simulink model "torqueBalancingYogaWithQPBlock2017a_"  (Simulink 8.9)
settings: Solver=FixedStepDiscrete  StartTime=0.0  StopTime="Config.SIMULATION_TIME "  FixedStep=Config.Ts  RelTol=1e-3  EnableMultiTasking=on
InitFcn:
  | cd(fileparts(which(bdroot)));
  | initTorqueBalancingYoga;
StopFcn:
  | cd(fileparts(which(bdroot)));
  | stopTorqueBalancingYoga;
undefined symbols (not defined in the file or in its folder): bVectorConstraints, Config, ConstraintsMatrix, Gain, Reg, ROBOT_DOF, ROBOT_DOF_FOR_SIMULINK, Sat, Sm
libraries: WBToolboxLibrary x90, simulink x4
(part 1 of 2)
settings Model: SuppressorTable=22 serialization::archive 11 0 6 0 0 0 1 0  Creator=daniele  LastModifiedBy=root
settings DataIOCC: SignalLoggingSaveFormat=Dataset
settings OptimizationCC: ExpressionDepthLimit=2147483647
settings DebuggingCC: SolverPrmCheckMsg=warning  AllowSymbolicDim=off
settings SFSimCC: SimParseCustomCode=off
settings RTWCC: GenCodeOnly=on  RetainRTWFile=on  BuildConfiguration=Debug  TargetLang=C++
settings GRTTargetCC: TargetLangStandard=C++03 (ISO)  GenerateFullHeader=off  CombineOutputUpdateFcns=on  MatFileLogging=off  MultiInstanceERTCode=on  CodeInterfacePackaging=C++ class  SupportNonFinite=off  GRTInterface=off
settings CPPComponent: GenerateDestructor=on  GenerateExternalIOAccessMethods=None  ParameterMemberVisibility=private  InternalMemberVisibility=private  GenerateParameterAccessMethods=None  GenerateInternalMemberAccessMethods=None  UseOperatorNewForModelRefRegistration=off

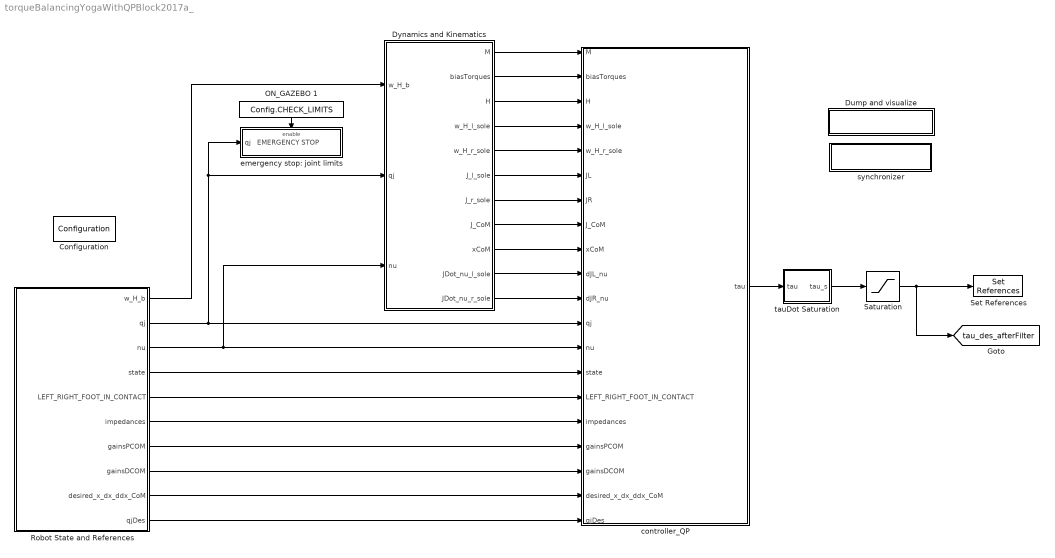
== system torqueBalancingYogaWithQPBlock2017a_ ==
  Configuration : WBToolboxLibrary/Utilities/Configuration  ConfigSource=Workspace  ConfigObject='WBTConfigRobot'
      settings: SourceProductName=Whole Body Toolbox
  Dump and visualize : Subsystem
      mask Display: disp('VISUALIZER')
  Dynamics and Kinematics : Subsystem
  ON_GAZEBO 1 : Constant  Value=Config.CHECK_LIMITS
  Robot State and References : Subsystem  Priority=-10
  Saturation : Saturate  UpperLimit=Sat.torque  LowerLimit=-Sat.torque
  Set References : WBToolboxLibrary/wholeBodyActuators/Set References  controlType=Torque  refSpeed=50
      settings: SourceProductName=Whole Body Toolbox
  controller_QP : Subsystem
  emergency stop: joint limits : Subsystem
  synchronizer : Subsystem
      mask Display: disp('SYNCHRONIZER')
  tauDot Saturation : Subsystem
  tag scope: tau_des_afterFilter=global
  wires:
  Saturation/1 -> [tau_des_afterFilter], Set References/1
  ON_GAZEBO 1/1 -> emergency stop: joint limits/Enable
  Dynamics and Kinematics/1(M) -> controller_QP/1(M)
  Dynamics and Kinematics/2(biasTorques) -> controller_QP/2(biasTorques)
  Dynamics and Kinematics/3(H) -> controller_QP/3("H ")
  Dynamics and Kinematics/4(w_H_l_sole) -> controller_QP/4(w_H_l_sole)
  Dynamics and Kinematics/5(w_H_r_sole) -> controller_QP/5(w_H_r_sole)
  Dynamics and Kinematics/6(J_l_sole) -> controller_QP/6(JL)
  Dynamics and Kinematics/7(J_r_sole) -> controller_QP/7(JR)
  Dynamics and Kinematics/8(J_CoM) -> controller_QP/8(J_CoM)
  Dynamics and Kinematics/9(xCoM) -> controller_QP/9(xCoM)
  Dynamics and Kinematics/10(JDot_nu_l_sole) -> controller_QP/10(dJL_nu)
  Dynamics and Kinematics/11(JDot_nu_r_sole) -> controller_QP/11(dJR_nu)
  Robot State and References/1(w_H_b) -> Dynamics and Kinematics/1(w_H_b)
  Robot State and References/2(qj) -> controller_QP/12(qj), emergency stop: joint limits/1(qj   EMERGENCY STOP), Dynamics and Kinematics/2(qj)
  Robot State and References/3(nu) -> controller_QP/13(nu), Dynamics and Kinematics/3(nu)
  Robot State and References/4(state) -> controller_QP/14(state)
  Robot State and References/5(LEFT_RIGHT_FOOT_IN_CONTACT) -> controller_QP/15(LEFT_RIGHT_FOOT_IN_CONTACT)
  Robot State and References/6(impedances) -> controller_QP/16(impedances)
  Robot State and References/7(gainsPCOM) -> controller_QP/17(gainsPCOM)
  Robot State and References/8(gainsDCOM) -> controller_QP/18(gainsDCOM)
  Robot State and References/9(desired_x_dx_ddx_CoM) -> controller_QP/19(desired_x_dx_ddx_CoM)
  Robot State and References/10(qjDes) -> controller_QP/20(qjDes)
  controller_QP/1("tau ") -> tauDot Saturation/1(tau)
  tauDot Saturation/1(tau_s) -> Saturation/1

== system torqueBalancingYogaWithQPBlock2017a_/Dump and visualize ==
  Logical Operator1 : Logic  Operator=OR  AllPortsSameDT=off  OutDataTypeStr=boolean
  ON_GAZEBO 3 : Constant  Value=Config.SCOPES_ALL
  ON_GAZEBO 4 : Constant  Value=Config.SCOPES_MAIN
  Visualizer : Subsystem
  wires:
  ON_GAZEBO 3/1 -> Logical Operator1/1
  ON_GAZEBO 4/1 -> Logical Operator1/2
  Logical Operator1/1 -> Visualizer/Enable
  [state] -> Visualizer/3(state)
  [CoM_error] -> Visualizer/5(CoM_Error)
  [f_QP] -> Visualizer/6(fDesQP)
  [f_noQP] -> Visualizer/8(fDesNoQP)
  [qj_des] -> Visualizer/4(qj_des)
  [w_H_b] -> Visualizer/2(w_H_b)
  [tau_des] -> Visualizer/1(tau_des)
  [CoM_des] -> Visualizer/7(CoM_des)
  [tau_des_afterFilter] -> Visualizer/9(tau_des_afterFilter)

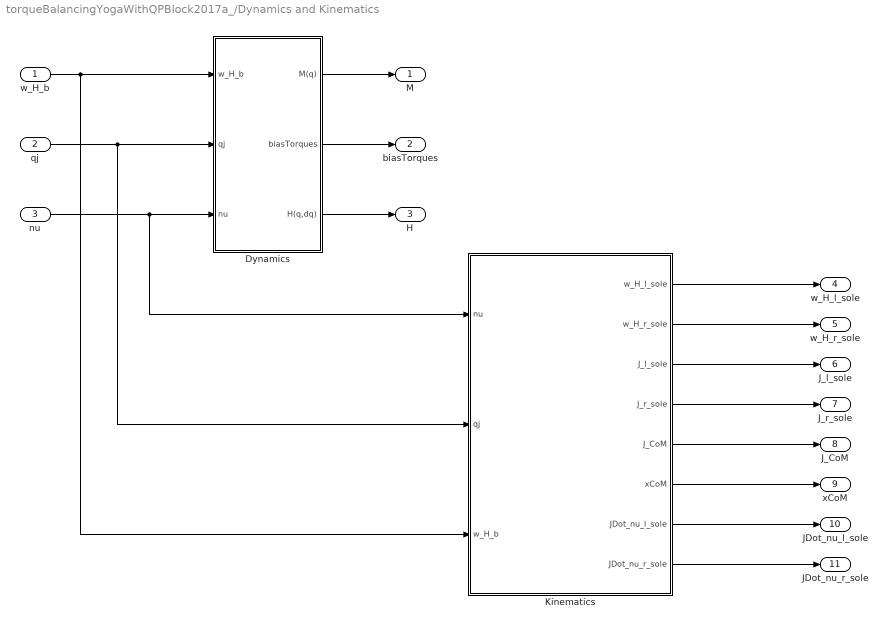
== system torqueBalancingYogaWithQPBlock2017a_/Dynamics and Kinematics ==
  w_H_b : Inport
  qj : Inport  Port=2
  nu : Inport  Port=3
  Dynamics : Subsystem
  Kinematics : Subsystem
  M : Outport
  biasTorques : Outport  Port=2
  H : Outport  Port=3
  w_H_l_sole : Outport  Port=4
  w_H_r_sole : Outport  Port=5
  J_l_sole : Outport  Port=6
  J_r_sole : Outport  Port=7
  J_CoM : Outport  Port=8
  xCoM : Outport  Port=9
  JDot_nu_l_sole : Outport  Port=10
  JDot_nu_r_sole : Outport  Port=11
  wires:
  w_H_b/1 -> Kinematics/3(w_H_b), Dynamics/1(w_H_b)
  qj/1 -> Dynamics/2(qj), Kinematics/2(qj)
  nu/1 -> Dynamics/3(nu), Kinematics/1(nu)
  Dynamics/1(M(q)) -> M/1
  Dynamics/2(biasTorques) -> biasTorques/1
  Dynamics/3(H(q,dq)) -> H/1
  Kinematics/7(JDot_nu_l_sole) -> JDot_nu_l_sole/1
  Kinematics/8(JDot_nu_r_sole) -> JDot_nu_r_sole/1
  Kinematics/4(J_r_sole) -> J_r_sole/1
  Kinematics/1(w_H_l_sole) -> w_H_l_sole/1
  Kinematics/3(J_l_sole) -> J_l_sole/1
  Kinematics/5(J_CoM) -> J_CoM/1
  Kinematics/6(xCoM) -> xCoM/1
  Kinematics/2(w_H_r_sole) -> w_H_r_sole/1

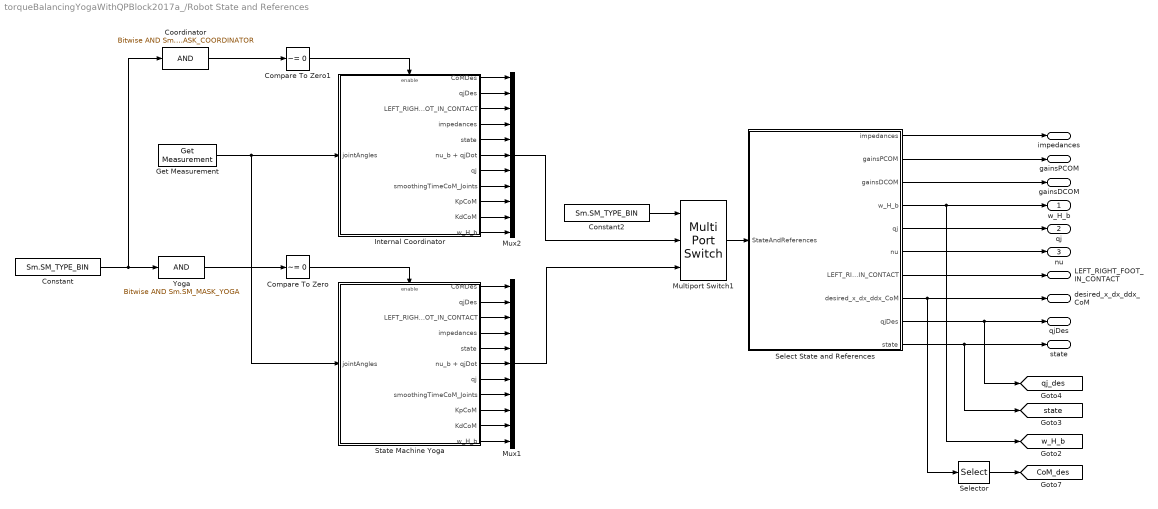
== system torqueBalancingYogaWithQPBlock2017a_/Robot State and References ==
  Compare To Zero : simulink/Logic and Bit Operations/Compare To Zero  relop=~=  OutDataTypeStr=boolean
  Compare To Zero1 : simulink/Logic and Bit Operations/Compare To Zero  relop=~=  OutDataTypeStr=boolean
  Constant : Constant  Priority=-10  Value=Sm.SM_TYPE_BIN  OutDataTypeStr=uint8
  Constant2 : Constant  Priority=-10  Value=Sm.SM_TYPE_BIN  OutDataTypeStr=uint8
  Coordinator : simulink/Logic and Bit Operations/Bitwise Operator  logicop=AND  UseBitMask=on  BitMask=Sm.SM_MASK_COORDINATOR  BitMaskRealWorld=Stored Integer
  Get Measurement : WBToolboxLibrary/wholeBodyStates/Get Measurement  measuredType=Joints Position
      settings: SourceProductName=Whole Body Toolbox
  Internal Coordinator : Subsystem
  Multiport Switch1 : MultiPortSwitch  DataPortOrder=Specify indices  DataPortIndices={1, 2}
  Mux1 : Mux  Inputs=11
  Mux2 : Mux  Inputs=11
  Select State and References : Subsystem
  Selector : Selector  NumberOfDimensions=2  InputPortWidth=3  IndexOptions=Index vector (dialog),Index vector (dialog)  Indices=[1 2 3],[1]  OutputSizes=1,1
  State Machine Yoga : Subsystem  Priority=-100
  Yoga : simulink/Logic and Bit Operations/Bitwise Operator  logicop=AND  UseBitMask=on  BitMask=Sm.SM_MASK_YOGA  BitMaskRealWorld=Stored Integer
  w_H_b : Outport
  qj : Outport  Port=2
  nu : Outport  Port=3
  state : Outport  Port=4
  LEFT_RIGHT_FOOT_IN_CONTACT : Outport  Port=5
  impedances : Outport  Port=6
  gainsPCOM : Outport  Port=7
  gainsDCOM : Outport  Port=8
  desired_x_dx_ddx_CoM : Outport  Port=9
  qjDes : Outport  Port=10
  tag scope: CoM_des=global, qj_des=global, state=global, w_H_b=global
  wires:
  Constant/1 -> Yoga/1, Coordinator/1
  State Machine Yoga/3(LEFT_RIGHT_FOOT_IN_CONTACT) -> Mux1/3
  State Machine Yoga/2(qjDes) -> Mux1/2
  State Machine Yoga/1(CoMDes) -> Mux1/1
  Internal Coordinator/1(CoMDes) -> Mux2/1
  Internal Coordinator/2(qjDes) -> Mux2/2
  Internal Coordinator/3(LEFT_RIGHT_FOOT_IN_CONTACT) -> Mux2/3
  State Machine Yoga/4(impedances) -> Mux1/4
  Internal Coordinator/4(impedances) -> Mux2/4
  State Machine Yoga/5(state) -> Mux1/5
  Internal Coordinator/5(state) -> Mux2/5
  Internal Coordinator/6(nu_b + qjDot) -> Mux2/6
  Internal Coordinator/7(qj) -> Mux2/7
  State Machine Yoga/6(nu_b + qjDot) -> Mux1/6
  State Machine Yoga/7(qj) -> Mux1/7
  Coordinator/1 -> Compare To Zero1/1
  Yoga/1 -> Compare To Zero/1
  Compare To Zero/1 -> State Machine Yoga/Enable
  Compare To Zero1/1 -> Internal Coordinator/Enable
  Internal Coordinator/8(smoothingTimeCoM_Joints) -> Mux2/8
  State Machine Yoga/8(smoothingTimeCoM_Joints) -> Mux1/8
  State Machine Yoga/9(KpCoM) -> Mux1/9
  State Machine Yoga/10(KdCoM) -> Mux1/10
  Internal Coordinator/9(KpCoM) -> Mux2/9
  Internal Coordinator/10(KdCoM) -> Mux2/10
  Constant2/1 -> Multiport Switch1/1
  Get Measurement/1 -> Internal Coordinator/1(jointAngles), State Machine Yoga/1(jointAngles)
  State Machine Yoga/11(w_H_b) -> Mux1/11
  Internal Coordinator/11(w_H_b) -> Mux2/11
  Mux2/1 -> Multiport Switch1/2
  Mux1/1 -> Multiport Switch1/3
  Multiport Switch1/1 -> Select State and References/1(StateAndReferences)
  Select State and References/1(impedances) -> impedances/1
  Select State and References/2(gainsPCOM) -> gainsPCOM/1
  Select State and References/3(gainsDCOM) -> gainsDCOM/1
  Select State and References/4(w_H_b) -> w_H_b/1, [w_H_b]
  Select State and References/5(qj) -> qj/1
  Select State and References/6(nu) -> nu/1
  Select State and References/7(LEFT_RIGHT_FOOT_IN_CONTACT) -> LEFT_RIGHT_FOOT_IN_CONTACT/1
  Select State and References/8(desired_x_dx_ddx_CoM) -> desired_x_dx_ddx_CoM/1, Selector/1
  Select State and References/9(qjDes) -> qjDes/1, [qj_des]
  Select State and References/10(state) -> state/1, [state]
  Selector/1 -> [CoM_des]

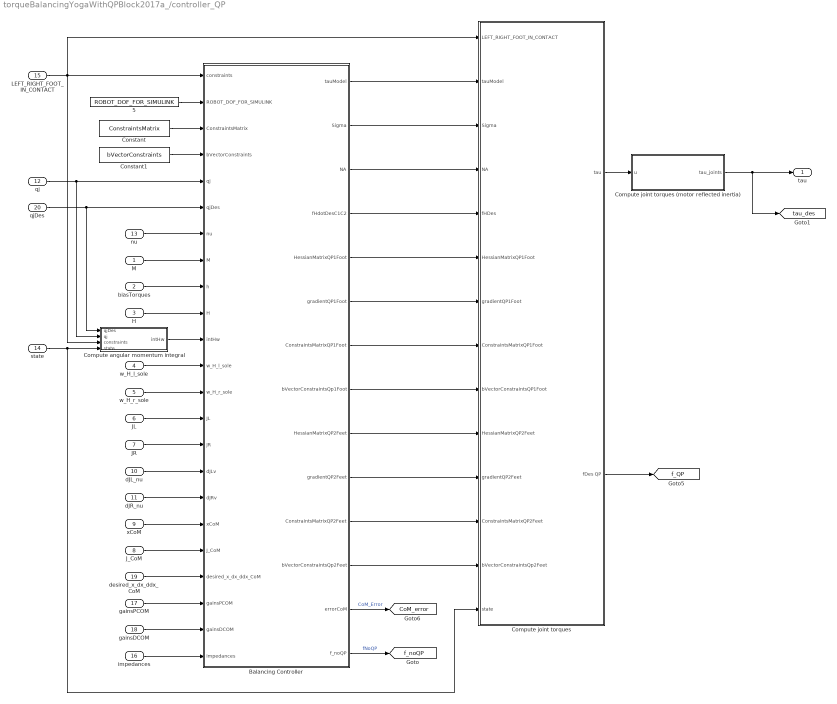
== system torqueBalancingYogaWithQPBlock2017a_/controller_QP ==
  M : Inport
  biasTorques : Inport  Port=2
  "H " : Inport  Port=3
  w_H_l_sole : Inport  Port=4
  w_H_r_sole : Inport  Port=5
  JL : Inport  Port=6
  JR : Inport  Port=7
  J_CoM : Inport  Port=8
  xCoM : Inport  Port=9
  dJL_nu : Inport  Port=10
  dJR_nu : Inport  Port=11
  qj : Inport  Port=12
  nu : Inport  Port=13
  state : Inport  Port=14
  LEFT_RIGHT_FOOT_IN_CONTACT : Inport  Port=15
  impedances : Inport  Port=16
  gainsPCOM : Inport  Port=17
  gainsDCOM : Inport  Port=18
  desired_x_dx_ddx_CoM : Inport  Port=19
  qjDes : Inport  Port=20
  "    5" : Constant  Value=ROBOT_DOF_FOR_SIMULINK
  "Balancing Controller " : MATLAB Function  TreatAsAtomicUnit=on
  Compute angular momentum integral : Subsystem
  Compute joint torques : Subsystem
  Compute joint torques (motor reflected inertia) : Subsystem
  Constant : Constant  Value=ConstraintsMatrix
  Constant1 : Constant  Value=bVectorConstraints
  "tau " : Outport
  tag scope: CoM_error=global, f_QP=global, f_noQP=global, tau_des=global
  wires:
  LEFT_RIGHT_FOOT_IN_CONTACT/1 -> "Balancing Controller "/1(constraints), Compute joint torques/1(LEFT_RIGHT_FOOT_IN_CONTACT), Compute angular momentum integral/3(constraints)
  qj/1 -> Compute angular momentum integral/2(qj), "Balancing Controller "/5(qj)
  qjDes/1 -> Compute angular momentum integral/1(qjDes), "Balancing Controller "/6(qjDes)
  M/1 -> "Balancing Controller "/8(M)
  biasTorques/1 -> "Balancing Controller "/9(h)
  desired_x_dx_ddx_CoM/1 -> "Balancing Controller "/20(desired_x_dx_ddx_CoM)
  impedances/1 -> "Balancing Controller "/23(impedances)
  "H "/1 -> "Balancing Controller "/10(H)
  "    5"/1 -> "Balancing Controller "/2(ROBOT_DOF_FOR_SIMULINK)
  Constant/1 -> "Balancing Controller "/3(ConstraintsMatrix)
  Constant1/1 -> "Balancing Controller "/4(bVectorConstraints)
  nu/1 -> "Balancing Controller "/7(nu)
  gainsPCOM/1 -> "Balancing Controller "/21(gainsPCOM)
  gainsDCOM/1 -> "Balancing Controller "/22(gainsDCOM)
  w_H_r_sole/1 -> "Balancing Controller "/13(w_H_r_sole)
  w_H_l_sole/1 -> "Balancing Controller "/12(w_H_l_sole)
  JL/1 -> "Balancing Controller "/14(JL)
  JR/1 -> "Balancing Controller "/15(JR)
  Compute angular momentum integral/1(intHw) -> "Balancing Controller "/11(intHw)
  dJL_nu/1 -> "Balancing Controller "/16(dJLv)
  dJR_nu/1 -> "Balancing Controller "/17(dJRv)
  J_CoM/1 -> "Balancing Controller "/19(J_CoM)
  xCoM/1 -> "Balancing Controller "/18(xCoM)
  state/1 -> Compute angular momentum integral/4(state), Compute joint torques/14(state)
  Compute joint torques/1("tau ") -> Compute joint torques (motor reflected inertia)/1(u)
  "Balancing Controller "/1(tauModel) -> Compute joint torques/2(tauModel)
  "Balancing Controller "/2(Sigma) -> Compute joint torques/3(Sigma)
  "Balancing Controller "/3(NA) -> Compute joint torques/4(NA)
  "Balancing Controller "/4(fHdotDesC1C2) -> Compute joint torques/5(fHDes)
  "Balancing Controller "/5(HessianMatrixQP1Foot) -> Compute joint torques/6(HessianMatrixQP1Foot)
  "Balancing Controller "/6(gradientQP1Foot) -> Compute joint torques/7(gradientQP1Foot)
  "Balancing Controller "/7(ConstraintsMatrixQP1Foot) -> Compute joint torques/8(ConstraintsMatrixQP1Foot)
  "Balancing Controller "/8(bVectorConstraintsQp1Foot) -> Compute joint torques/9(bVectorConstraintsQP1Foot)
  "Balancing Controller "/9(HessianMatrixQP2Feet) -> Compute joint torques/10(HessianMatrixQP2Feet)
  "Balancing Controller "/10(gradientQP2Feet) -> Compute joint torques/11(gradientQP2Feet)
  "Balancing Controller "/11(ConstraintsMatrixQP2Feet) -> Compute joint torques/12(ConstraintsMatrixQP2Feet)
  "Balancing Controller "/12(bVectorConstraintsQp2Feet) -> Compute joint torques/13(bVectorConstraintsQp2Feet)
  "Balancing Controller "/13(errorCoM) -> [CoM_error]  "CoM_Error"
  Compute joint torques/2(fDes QP) -> [f_QP]
  "Balancing Controller "/14(f_noQP) -> [f_noQP]  "fNoQP"
  Compute joint torques (motor reflected inertia)/1(tau_joints) -> "tau "/1, [tau_des]

== system torqueBalancingYogaWithQPBlock2017a_/emergency stop: joint limits ==
  qj   EMERGENCY STOP : Inport
  Enable : EnablePort
  Assertion : Assertion
  Get Limits : WBToolboxLibrary/wholeBodyStates/Get Limits  limitsSource=ControlBoard  limitsType=Position
      settings: SourceProductName=Whole Body Toolbox
  MATLAB Function : MATLAB Function  TreatAsAtomicUnit=on
  index1 : Constant  Value=0.01  VectorParams1D=off
  wires:
  Get Limits/1 -> MATLAB Function/1(umin)
  Get Limits/2 -> MATLAB Function/2(umax)
  index1/1 -> MATLAB Function/4(tol)
  qj   EMERGENCY STOP/1 -> MATLAB Function/3(u)
  MATLAB Function/1(inRange) -> Assertion/1

== system torqueBalancingYogaWithQPBlock2017a_/synchronizer ==
  GAZEBO_SYNCHRONIZER : Subsystem
  Logical Operator : Logic  Operator=NOT  AllPortsSameDT=off  OutDataTypeStr=boolean
  "ON_GAZEBO " : Constant  Value=Config.ON_GAZEBO
  REAL_TIME_SYNC : Subsystem
  wires:
  Logical Operator/1 -> REAL_TIME_SYNC/Enable
  "ON_GAZEBO "/1 -> GAZEBO_SYNCHRONIZER/Enable, Logical Operator/1

== system torqueBalancingYogaWithQPBlock2017a_/tauDot Saturation ==
  tau : Inport
  Constant : Constant  Value=Config.SATURATE_TORQUE_DERIVATIVE
  Saturate the Torque Derivative : MATLAB Function  TreatAsAtomicUnit=on
  Switch : Switch  Criteria=u2 > Threshold
  "holder " : WBToolboxLibrary/Utilities/holder 
      settings: SourceProductName=Whole Body Toolbox
  tau_s : Outport
  wires:
  Switch/1 -> tau_s/1
  Constant/1 -> Switch/2
  tau/1 -> "holder "/1, Saturate the Torque Derivative/1(u), Switch/3
  Saturate the Torque Derivative/1(uSat) -> Switch/1
  "holder "/1 -> Saturate the Torque Derivative/2(u_0)

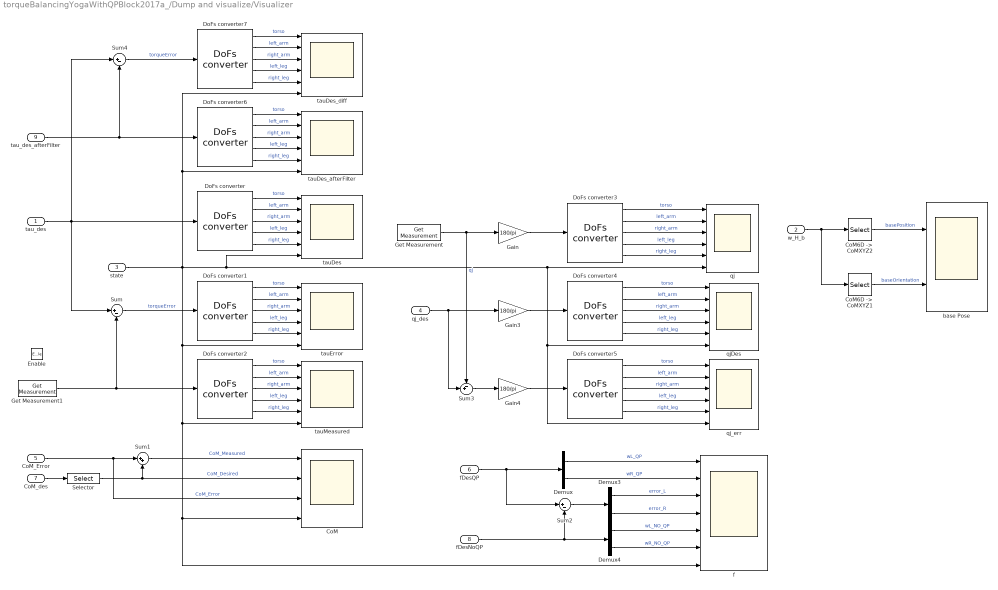
== system torqueBalancingYogaWithQPBlock2017a_/Dump and visualize/Visualizer ==
  tau_des : Inport
  w_H_b : Inport  Port=2
  state : Inport  Port=3
  qj_des : Inport  Port=4
  CoM_Error : Inport  Port=5
  fDesQP : Inport  Port=6
  CoM_des : Inport  Port=7
  fDesNoQP : Inport  Port=8
  tau_des_afterFilter : Inport  Port=9
  Enable : EnablePort
  CoM : Scope  NumInputPorts=4
  "CoM6D ->  CoMXYZ1" : Selector  NumberOfDimensions=2  InputPortWidth=7  IndexOptions=Index vector (dialog),Index vector (dialog)  Indices=[1 2 3],[1 2 3]  OutputSizes=1,1
  "CoM6D ->  CoMXYZ2" : Selector  NumberOfDimensions=2  InputPortWidth=7  IndexOptions=Index vector (dialog),Index vector (dialog)  Indices=[1 2 3],[4]  OutputSizes=1,1
  Demux : Demux  Outputs=2
  Demux3 : Demux  Outputs=2
  Demux4 : Demux  Outputs=2
  DoFs converter{,1..7} (8 alike) : WBToolboxLibrary/Utilities/DoFs converter  yarp2WBIOption=From YARP to WBI
      settings: SourceProductName=Whole Body Toolbox
  Gain : Gain  Gain=180/pi
  Gain3 : Gain  Gain=180/pi
  Gain4 : Gain  Gain=180/pi
  Get Measurement : WBToolboxLibrary/wholeBodyStates/Get Measurement  measuredType=Joints Position
      settings: SourceProductName=Whole Body Toolbox
  Get Measurement1 : WBToolboxLibrary/wholeBodyStates/Get Measurement  measuredType=Joints Torque
      settings: SourceProductName=Whole Body Toolbox
  Selector : Selector  NumberOfDimensions=2  IndexOptions=Index vector (dialog),Index vector (dialog)  Indices=[1:3],1  OutputSizes=1,1
  Sum : Sum  Inputs=|+-
  Sum1 : Sum  Inputs=|++
  Sum2 : Sum  Inputs=|+-
  Sum3 : Sum  Inputs=-+|
  Sum4 : Sum  Inputs=|+-
  base Pose : Scope  NumInputPorts=2
  f : Scope  NumInputPorts=7
  qj : Scope  NumInputPorts=6
  qjDes : Scope  NumInputPorts=6
  qj_err : Scope  NumInputPorts=6
  tauDes : Scope  NumInputPorts=6
  tauDes_afterFilter : Scope  NumInputPorts=6
  tauDes_diff : Scope  NumInputPorts=6
  tauError : Scope  NumInputPorts=6
  tauMeasured : Scope  NumInputPorts=6
  wires:
  CoM_Error/1 -> Sum1/1, CoM/3  "CoM_Error"
  CoM_des/1 -> Selector/1
  Gain/1 -> DoFs converter3/1
  Sum1/1 -> CoM/1  "CoM_Measured"
  Get Measurement/1 -> Gain/1, Sum3/1  "qj"
  DoFs converter3/5 -> qj/5  "right_leg"
  DoFs converter3/1 -> qj/1  "torso"
  DoFs converter3/2 -> qj/2  "left_arm"
  DoFs converter3/4 -> qj/4  "left_leg"
  fDesQP/1 -> Sum2/1, Demux/1
  DoFs converter3/3 -> qj/3  "right_arm"
  Sum2/1 -> Demux3/1
  fDesNoQP/1 -> Sum2/2, Demux4/1
  Get Measurement1/1 -> DoFs converter2/1, Sum/2
  DoFs converter/5 -> tauDes/5  "right_leg"
  DoFs converter/1 -> tauDes/1  "torso"
  DoFs converter/2 -> tauDes/2  "left_arm"
  DoFs converter/4 -> tauDes/4  "left_leg"
  DoFs converter/3 -> tauDes/3  "right_arm"
  DoFs converter1/5 -> tauError/5  "right_leg"
  DoFs converter1/1 -> tauError/1  "torso"
  DoFs converter1/2 -> tauError/2  "left_arm"
  DoFs converter1/4 -> tauError/4  "left_leg"
  DoFs converter1/3 -> tauError/3  "right_arm"
  Sum/1 -> DoFs converter1/1  "torqueError"
  DoFs converter2/5 -> tauMeasured/5  "right_leg"
  DoFs converter2/1 -> tauMeasured/1  "torso"
  DoFs converter2/2 -> tauMeasured/2  "left_arm"
  DoFs converter2/4 -> tauMeasured/4  "left_leg"
  DoFs converter2/3 -> tauMeasured/3  "right_arm"
  qj_des/1 -> Sum3/2, Gain3/1
  Gain3/1 -> DoFs converter4/1
  DoFs converter4/5 -> qjDes/5  "right_leg"
  DoFs converter4/1 -> qjDes/1  "torso"
  DoFs converter4/2 -> qjDes/2  "left_arm"
  DoFs converter4/4 -> qjDes/4  "left_leg"
  DoFs converter4/3 -> qjDes/3  "right_arm"
  Gain4/1 -> DoFs converter5/1
  DoFs converter5/5 -> qj_err/5  "right_leg"
  DoFs converter5/1 -> qj_err/1  "torso"
  DoFs converter5/2 -> qj_err/2  "left_arm"
  DoFs converter5/4 -> qj_err/4  "left_leg"
  DoFs converter5/3 -> qj_err/3  "right_arm"
  Sum3/1 -> Gain4/1
  Selector/1 -> Sum1/2, CoM/2  "CoM_Desired"
  Demux/1 -> f/1  "wL_QP"
  Demux/2 -> f/2  "wR_QP"
  Demux3/1 -> f/3  "error_L"
  Demux3/2 -> f/4  "error_R"
  Demux4/1 -> f/5  "wL_NO_QP"
  Demux4/2 -> f/6  "wR_NO_QP"
  w_H_b/1 -> "CoM6D ->  CoMXYZ1"/1, "CoM6D ->  CoMXYZ2"/1
  "CoM6D ->  CoMXYZ2"/1 -> base Pose/1  "basePosition"
  "CoM6D ->  CoMXYZ1"/1 -> base Pose/2  "baseOrientation"
  DoFs converter6/4 -> tauDes_afterFilter/4  "left_leg"
  DoFs converter6/5 -> tauDes_afterFilter/5  "right_leg"
  DoFs converter6/2 -> tauDes_afterFilter/2  "left_arm"
  DoFs converter6/1 -> tauDes_afterFilter/1  "torso"
  DoFs converter6/3 -> tauDes_afterFilter/3  "right_arm"
  tau_des_afterFilter/1 -> Sum4/2, DoFs converter6/1
  Sum4/1 -> DoFs converter7/1  "torqueError"
  tau_des/1 -> Sum4/1, DoFs converter/1, Sum/1
  DoFs converter7/5 -> tauDes_diff/5  "right_leg"
  state/1 -> tauDes_diff/6, tauDes_afterFilter/6, qj_err/6, qjDes/6, qj/6, tauDes/6, f/7, CoM/4, tauMeasured/6, tauError/6
  DoFs converter7/3 -> tauDes_diff/3  "right_arm"
  DoFs converter7/2 -> tauDes_diff/2  "left_arm"
  DoFs converter7/4 -> tauDes_diff/4  "left_leg"
  DoFs converter7/1 -> tauDes_diff/1  "torso"

== system torqueBalancingYogaWithQPBlock2017a_/Dynamics and Kinematics/Dynamics ==
  w_H_b : Inport
  qj : Inport  Port=2
  nu : Inport  Port=3
  Add motors reflected inertias : Subsystem
  Centroidal Momentum : WBToolboxLibrary/wholeBodyModel/Dynamics/Centroidal Momentum
      settings: SourceProductName=Whole Body Toolbox
  "CoM6D ->  CoMXYZ1" : Selector  InputPortWidth=6+ROBOT_DOF  IndexOptions=Index vector (dialog)  Indices=[7:6+ROBOT_DOF]  OutputSizes=1
  "CoM6D ->  CoMXYZ2" : Selector  InputPortWidth=6+ROBOT_DOF  IndexOptions=Index vector (dialog)  Indices=[1 2 3 4 5 6]  OutputSizes=1
  Get Bias Forces : WBToolboxLibrary/wholeBodyModel/Dynamics/Get Bias Forces
      settings: SourceProductName=Whole Body Toolbox
  Mass Matrix : WBToolboxLibrary/wholeBodyModel/Dynamics/Mass Matrix
      settings: SourceProductName=Whole Body Toolbox
  M(q) : Outport
  biasTorques : Outport  Port=2
  H(q,dq) : Outport  Port=3
  wires:
  Centroidal Momentum/1 -> H(q,dq)/1
  Get Bias Forces/1 -> biasTorques/1
  w_H_b/1 -> Centroidal Momentum/1, Get Bias Forces/1, Mass Matrix/1
  qj/1 -> Centroidal Momentum/2, Get Bias Forces/2, Mass Matrix/2
  "CoM6D ->  CoMXYZ2"/1 -> Centroidal Momentum/3, Get Bias Forces/3
  "CoM6D ->  CoMXYZ1"/1 -> Centroidal Momentum/4, Get Bias Forces/4
  nu/1 -> "CoM6D ->  CoMXYZ1"/1, "CoM6D ->  CoMXYZ2"/1
  Mass Matrix/1 -> Add motors reflected inertias/1(M)
  Add motors reflected inertias/1(M_with_motor_inertia) -> M(q)/1

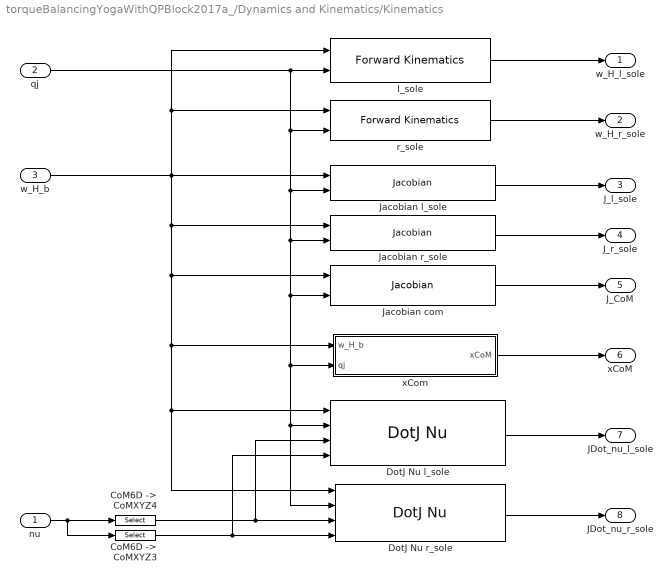
== system torqueBalancingYogaWithQPBlock2017a_/Dynamics and Kinematics/Kinematics ==
  nu : Inport
  qj : Inport  Port=2
  w_H_b : Inport  Port=3
  "CoM6D ->  CoMXYZ3" : Selector  InputPortWidth=6+ROBOT_DOF  IndexOptions=Index vector (dialog)  Indices=[7:6+ROBOT_DOF]  OutputSizes=1
  "CoM6D ->  CoMXYZ4" : Selector  InputPortWidth=6+ROBOT_DOF  IndexOptions=Index vector (dialog)  Indices=[1 2 3 4 5 6]  OutputSizes=1
  "DotJ Nu l_sole " : WBToolboxLibrary/wholeBodyModel/Jacobians/DotJ Nu  frameName=Frames.LEFT_FOOT
      settings: SourceProductName=Whole Body Toolbox
  "DotJ Nu r_sole   " : WBToolboxLibrary/wholeBodyModel/Jacobians/DotJ Nu  frameName=Frames.RIGHT_FOOT
      settings: SourceProductName=Whole Body Toolbox
  Jacobian com : WBToolboxLibrary/wholeBodyModel/Jacobians/Jacobian  frameName=Frames.COM
      settings: SourceProductName=Whole Body Toolbox
  Jacobian l_sole : WBToolboxLibrary/wholeBodyModel/Jacobians/Jacobian  frameName=Frames.LEFT_FOOT
      settings: SourceProductName=Whole Body Toolbox
  Jacobian r_sole : WBToolboxLibrary/wholeBodyModel/Jacobians/Jacobian  frameName=Frames.RIGHT_FOOT
      settings: SourceProductName=Whole Body Toolbox
  l_sole : WBToolboxLibrary/wholeBodyModel/Kinematics/Forward Kinematics  frameName=Frames.LEFT_FOOT
      settings: SourceProductName=Whole Body Toolbox
  r_sole : WBToolboxLibrary/wholeBodyModel/Kinematics/Forward Kinematics  frameName=Frames.RIGHT_FOOT
      settings: SourceProductName=Whole Body Toolbox
  xCom : Subsystem
  w_H_l_sole : Outport
  w_H_r_sole : Outport  Port=2
  J_l_sole : Outport  Port=3
  J_r_sole : Outport  Port=4
  J_CoM : Outport  Port=5
  xCoM : Outport  Port=6
  JDot_nu_l_sole : Outport  Port=7
  JDot_nu_r_sole : Outport  Port=8
  wires:
  "CoM6D ->  CoMXYZ3"/1 -> "DotJ Nu r_sole   "/4, "DotJ Nu l_sole "/4
  "CoM6D ->  CoMXYZ4"/1 -> "DotJ Nu r_sole   "/3, "DotJ Nu l_sole "/3
  nu/1 -> "CoM6D ->  CoMXYZ3"/1, "CoM6D ->  CoMXYZ4"/1
  w_H_b/1 -> Jacobian com/1, "DotJ Nu l_sole "/1, "DotJ Nu r_sole   "/1, xCom/1(w_H_b), Jacobian r_sole/1, Jacobian l_sole/1, r_sole/1, l_sole/1
  qj/1 -> Jacobian com/2, xCom/2(qj), "DotJ Nu r_sole   "/2, "DotJ Nu l_sole "/2, Jacobian r_sole/2, Jacobian l_sole/2, r_sole/2, l_sole/2
  l_sole/1 -> w_H_l_sole/1
  r_sole/1 -> w_H_r_sole/1
  Jacobian l_sole/1 -> J_l_sole/1
  Jacobian r_sole/1 -> J_r_sole/1
  Jacobian com/1 -> J_CoM/1
  xCom/1(xCoM) -> xCoM/1
  "DotJ Nu l_sole "/1 -> JDot_nu_l_sole/1
  "DotJ Nu r_sole   "/1 -> JDot_nu_r_sole/1

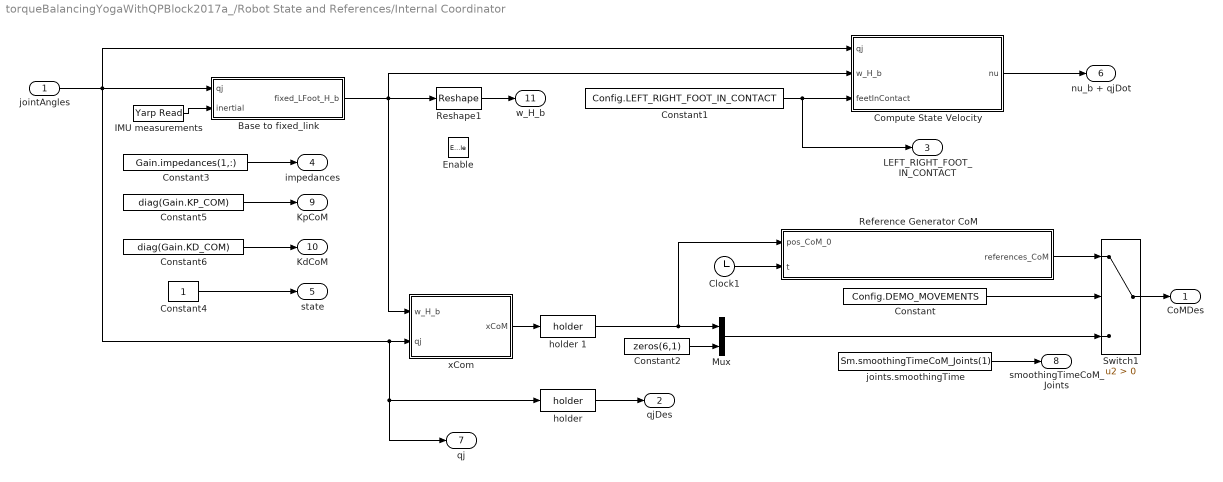
== system torqueBalancingYogaWithQPBlock2017a_/Robot State and References/Internal Coordinator ==
  jointAngles : Inport
  Enable : EnablePort
  Base to fixed_link : Subsystem
  Clock1 : Clock
  Compute State Velocity : Subsystem
  Constant : Constant  Value=Config.DEMO_MOVEMENTS
  Constant1 : Constant  Value=Config.LEFT_RIGHT_FOOT_IN_CONTACT
  Constant2 : Constant  Value=zeros(6,1)
  Constant3 : Constant  Value=Gain.impedances(1,:)
  Constant4 : Constant
  Constant5 : Constant  Value=diag(Gain.KP_COM)
  Constant6 : Constant  Value=diag(Gain.KD_COM)
  IMU measurements : WBToolboxLibrary/Utilities/Yarp Read  portName=Ports.IMU  signalSize=12  timeout=0.5  blocking=off  timestamp=off  autoconnect=on  errorOnConnection=on
      settings: SourceProductName=Whole Body Toolbox
  Mux : Mux  Inputs=2
  Reference Generator CoM : MATLAB Function  TreatAsAtomicUnit=on
  Reshape1 : Reshape  OutputDimensions=[4;4]
  Switch1 : Switch  Criteria=u2 > Threshold
  "holder " : WBToolboxLibrary/Utilities/holder 
      settings: SourceProductName=Whole Body Toolbox
  holder 1 : WBToolboxLibrary/Utilities/holder 
      settings: SourceProductName=Whole Body Toolbox
  joints.smoothingTime : Constant  Value=Sm.smoothingTimeCoM_Joints(1)
  xCom : Subsystem
  CoMDes : Outport
  qjDes : Outport  Port=2
  LEFT_RIGHT_FOOT_IN_CONTACT : Outport  Port=3
  impedances : Outport  Port=4
  state : Outport  Port=5
  nu_b + qjDot : Outport  Port=6
  qj : Outport  Port=7
  smoothingTimeCoM_Joints : Outport  Port=8
  KpCoM : Outport  Port=9
  KdCoM : Outport  Port=10
  w_H_b : Outport  Port=11
  wires:
  Constant/1 -> Switch1/2
  "holder "/1 -> qjDes/1
  Switch1/1 -> CoMDes/1
  Mux/1 -> Switch1/3
  Constant2/1 -> Mux/2
  Constant3/1 -> impedances/1
  Constant4/1 -> state/1
  Compute State Velocity/1(nu) -> nu_b + qjDot/1
  holder 1/1 -> Reference Generator CoM/1(pos_CoM_0), Mux/1
  Base to fixed_link/1(fixed_LFoot_H_b) -> Compute State Velocity/2(w_H_b), xCom/1(w_H_b), Reshape1/1
  xCom/1(xCoM) -> holder 1/1
  joints.smoothingTime/1 -> smoothingTimeCoM_Joints/1
  jointAngles/1 -> Compute State Velocity/1(qj), Base to fixed_link/1(qj), qj/1, "holder "/1, xCom/2(qj)
  Constant5/1 -> KpCoM/1
  Constant6/1 -> KdCoM/1
  Reshape1/1 -> w_H_b/1
  Constant1/1 -> Compute State Velocity/3("feetInContact "), LEFT_RIGHT_FOOT_IN_CONTACT/1
  IMU measurements/1 -> Base to fixed_link/2(inertial)
  Clock1/1 -> Reference Generator CoM/2(t)
  Reference Generator CoM/1(references_CoM) -> Switch1/1

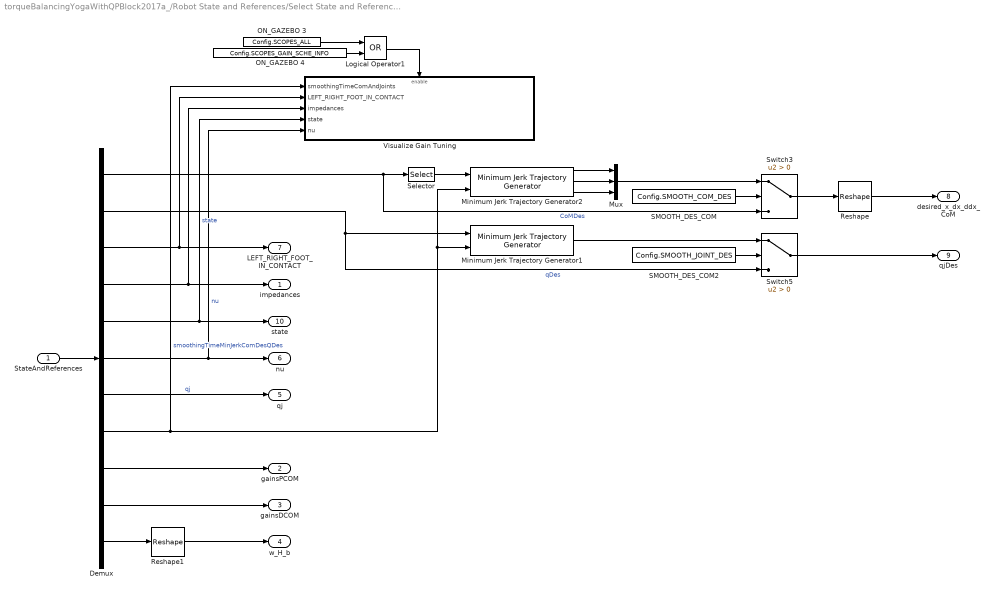
== system torqueBalancingYogaWithQPBlock2017a_/Robot State and References/Select State and References ==
  StateAndReferences : Inport
  Demux : Demux  Outputs=[9,ROBOT_DOF,2,ROBOT_DOF,1,ROBOT_DOF+6,ROBOT_DOF,1,3,3,16]
  Logical Operator1 : Logic  Operator=OR  AllPortsSameDT=off  OutDataTypeStr=boolean
  Minimum Jerk Trajectory Generator1 : WBToolboxLibrary/Utilities/Minimum Jerk Trajectory Generator  externalSettlingTime=on  settlingTime=1  sampleTime=Config.Ts  resetOnSettlingTime=off  firstDerivatives=off  secondDerivatives=off  explicitInitialValue=off
      settings: SourceProductName=Whole Body Toolbox
  Minimum Jerk Trajectory Generator2 : WBToolboxLibrary/Utilities/Minimum Jerk Trajectory Generator  externalSettlingTime=on  settlingTime=0  sampleTime=Config.Ts  resetOnSettlingTime=off  firstDerivatives=on  secondDerivatives=on  explicitInitialValue=off
      settings: SourceProductName=Whole Body Toolbox
  Mux : Mux  Inputs=3
  ON_GAZEBO 3 : Constant  Value=Config.SCOPES_ALL
  ON_GAZEBO 4 : Constant  Value=Config.SCOPES_GAIN_SCHE_INFO
  Reshape : Reshape  OutputDimensionality=Customize  OutputDimensions=[3,3]
  Reshape1 : Reshape  OutputDimensionality=Customize  OutputDimensions=[4;4]
  SMOOTH_DES_COM : Constant  Value=Config.SMOOTH_COM_DES
  SMOOTH_DES_COM2 : Constant  Value=Config.SMOOTH_JOINT_DES
  Selector : Selector  InputPortWidth=9  IndexOptions=Index vector (dialog)  Indices=[1 2 3]  OutputSizes=1
  Switch3 : Switch  Criteria=u2 > Threshold
  Switch5 : Switch  Criteria=u2 > Threshold
  "Visualize Gain Tuning  " : Subsystem
  impedances : Outport
  gainsPCOM : Outport  Port=2
  gainsDCOM : Outport  Port=3
  w_H_b : Outport  Port=4
  qj : Outport  Port=5
  nu : Outport  Port=6
  LEFT_RIGHT_FOOT_IN_CONTACT : Outport  Port=7
  desired_x_dx_ddx_CoM : Outport  Port=8
  qjDes : Outport  Port=9
  state : Outport  Port=10
  wires:
  Reshape/1 -> desired_x_dx_ddx_CoM/1
  Minimum Jerk Trajectory Generator2/1 -> Mux/1
  Minimum Jerk Trajectory Generator2/2 -> Mux/2
  Switch3/1 -> Reshape/1
  Minimum Jerk Trajectory Generator2/3 -> Mux/3
  SMOOTH_DES_COM/1 -> Switch3/2
  SMOOTH_DES_COM2/1 -> Switch5/2
  Switch5/1 -> qjDes/1
  Demux/7 -> qj/1  "qj"
  Demux/11 -> Reshape1/1
  Demux/5 -> "Visualize Gain Tuning  "/4(state), state/1  "state"
  Demux/8 -> Minimum Jerk Trajectory Generator2/2, Minimum Jerk Trajectory Generator1/2, "Visualize Gain Tuning  "/1(smoothingTimeComAndJoints)  "smoothingTimeMinJerkComDesQDes"
  Mux/1 -> Switch3/1
  Selector/1 -> Minimum Jerk Trajectory Generator2/1
  Demux/2 -> Switch5/3, Minimum Jerk Trajectory Generator1/1  "qDes"
  Minimum Jerk Trajectory Generator1/1 -> Switch5/1
  Demux/6 -> "Visualize Gain Tuning  "/5(nu), nu/1  "nu"
  StateAndReferences/1 -> Demux/1
  Demux/4 -> "Visualize Gain Tuning  "/3(impedances), impedances/1
  Demux/3 -> "Visualize Gain Tuning  "/2(LEFT_RIGHT_FOOT_IN_CONTACT), LEFT_RIGHT_FOOT_IN_CONTACT/1
  Demux/9 -> gainsPCOM/1
  Demux/10 -> gainsDCOM/1
  Demux/1 -> Switch3/3, Selector/1  "CoMDes"
  Reshape1/1 -> w_H_b/1
  ON_GAZEBO 4/1 -> Logical Operator1/2
  ON_GAZEBO 3/1 -> Logical Operator1/1
  Logical Operator1/1 -> "Visualize Gain Tuning  "/Enable

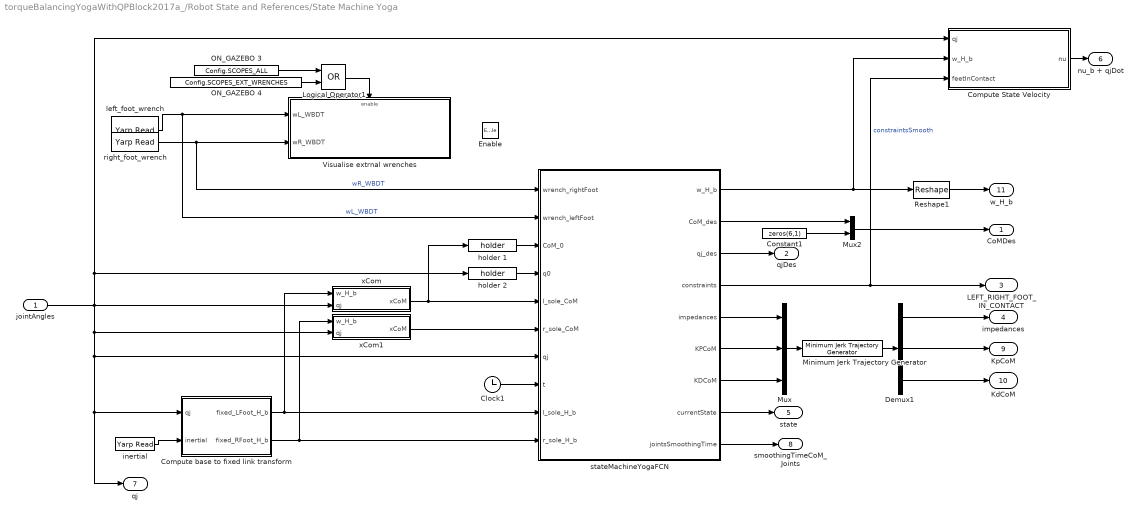
== system torqueBalancingYogaWithQPBlock2017a_/Robot State and References/State Machine Yoga ==
  jointAngles : Inport
  Enable : EnablePort
  Clock1 : Clock
  Compute State Velocity : Subsystem
  Compute base to fixed link transform : Subsystem
  Constant1 : Constant  Value=zeros(6,1)
  Demux1 : Demux  Outputs=[ROBOT_DOF,3,3]
  Logical Operator1 : Logic  Operator=OR  AllPortsSameDT=off  OutDataTypeStr=boolean
  Minimum Jerk Trajectory Generator : WBToolboxLibrary/Utilities/Minimum Jerk Trajectory Generator  externalSettlingTime=off  settlingTime=Gain.SmoothingTimeGainScheduling  sampleTime=Config.Ts  resetOnSettlingTime=off  firstDerivatives=off  secondDerivatives=off  explicitInitialValue=off
      settings: SourceProductName=Whole Body Toolbox
  Mux : Mux  Inputs=3
  Mux2 : Mux  Inputs=2
  ON_GAZEBO 3 : Constant  Value=Config.SCOPES_ALL
  ON_GAZEBO 4 : Constant  Value=Config.SCOPES_EXT_WRENCHES
  Reshape1 : Reshape  OutputDimensions=[4;4]
  "Visualise extrnal wrenches  " : Subsystem
  holder 1 : WBToolboxLibrary/Utilities/holder 
      settings: SourceProductName=Whole Body Toolbox
  holder 2 : WBToolboxLibrary/Utilities/holder 
      settings: SourceProductName=Whole Body Toolbox
  inertial : WBToolboxLibrary/Utilities/Yarp Read  portName=Ports.IMU  signalSize=12  timeout=0.5  blocking=off  timestamp=off  autoconnect=on  errorOnConnection=off
      settings: SourceProductName=Whole Body Toolbox
  left_foot_wrench : WBToolboxLibrary/Utilities/Yarp Read  portName=Ports.WBD_LEFTLEG_EE  signalSize=6  timeout=0.5  blocking=off  timestamp=off  autoconnect=on  errorOnConnection=on
      settings: SourceProductName=Whole Body Toolbox
  right_foot_wrench : WBToolboxLibrary/Utilities/Yarp Read  portName=Ports.WBD_RIGHTLEG_EE  signalSize=6  timeout=0.5  blocking=off  timestamp=off  autoconnect=on  errorOnConnection=on
      settings: SourceProductName=Whole Body Toolbox
  stateMachineYogaFCN : MATLAB Function  TreatAsAtomicUnit=on
  xCom : Subsystem
  xCom1 : Subsystem
  CoMDes : Outport
  qjDes : Outport  Port=2
  LEFT_RIGHT_FOOT_IN_CONTACT : Outport  Port=3
  impedances : Outport  Port=4
  state : Outport  Port=5
  nu_b + qjDot : Outport  Port=6
  qj : Outport  Port=7
  smoothingTimeCoM_Joints : Outport  Port=8
  KpCoM : Outport  Port=9
  KdCoM : Outport  Port=10
  w_H_b : Outport  Port=11
  wires:
  right_foot_wrench/1 -> "Visualise extrnal wrenches  "/2(wR_WBDT), stateMachineYogaFCN/1(wrench_rightFoot)  "wR_WBDT"
  xCom/1(xCoM) -> stateMachineYogaFCN/5(l_sole_CoM), holder 1/1
  holder 1/1 -> stateMachineYogaFCN/3(CoM_0)
  holder 2/1 -> stateMachineYogaFCN/4(q0)
  Clock1/1 -> stateMachineYogaFCN/8(t)
  stateMachineYogaFCN/3(qj_des) -> qjDes/1
  stateMachineYogaFCN/2(CoM_des) -> Mux2/1
  Mux2/1 -> CoMDes/1
  Constant1/1 -> Mux2/2
  stateMachineYogaFCN/8(currentState) -> state/1
  stateMachineYogaFCN/4(constraints) -> LEFT_RIGHT_FOOT_IN_CONTACT/1, Compute State Velocity/3("feetInContact ")  "constraintsSmooth"
  left_foot_wrench/1 -> "Visualise extrnal wrenches  "/1(wL_WBDT), stateMachineYogaFCN/2(wrench_leftFoot)  "wL_WBDT"
  stateMachineYogaFCN/1(w_H_b) -> Compute State Velocity/2(w_H_b), Reshape1/1
  xCom1/1(xCoM) -> stateMachineYogaFCN/6(r_sole_CoM)
  Compute State Velocity/1(nu) -> nu_b + qjDot/1
  stateMachineYogaFCN/9(jointsSmoothingTime) -> smoothingTimeCoM_Joints/1
  Logical Operator1/1 -> "Visualise extrnal wrenches  "/Enable
  ON_GAZEBO 3/1 -> Logical Operator1/1
  ON_GAZEBO 4/1 -> Logical Operator1/2
  stateMachineYogaFCN/6(KPCoM) -> Mux/2
  Demux1/3 -> KdCoM/1
  stateMachineYogaFCN/7(KDCoM) -> Mux/3
  stateMachineYogaFCN/5(impedances) -> Mux/1
  Mux/1 -> Minimum Jerk Trajectory Generator/1
  Minimum Jerk Trajectory Generator/1 -> Demux1/1
  Demux1/1 -> impedances/1
  Demux1/2 -> KpCoM/1
  jointAngles/1 -> xCom/2(qj), Compute State Velocity/1(qj), holder 2/1, stateMachineYogaFCN/7(qj), qj/1, Compute base to fixed link transform/1(qj), xCom1/2(qj)
  Compute base to fixed link transform/1(fixed_LFoot_H_b) -> stateMachineYogaFCN/9(l_sole_H_b), xCom/1(w_H_b)
  Compute base to fixed link transform/2(fixed_RFoot_H_b) -> stateMachineYogaFCN/10(r_sole_H_b), xCom1/1(w_H_b)
  inertial/1 -> Compute base to fixed link transform/2(inertial)
  Reshape1/1 -> w_H_b/1

== system torqueBalancingYogaWithQPBlock2017a_/controller_QP/Compute angular momentum integral ==
  qjDes : Inport
  qj : Inport  Port=2
  constraints : Inport  Port=3
  state : Inport  Port=4
  Centroidal Momentum : WBToolboxLibrary/wholeBodyModel/Dynamics/Centroidal Momentum
      settings: SourceProductName=Whole Body Toolbox
  Compute base to fixed link transform : Subsystem
  Jacobian : WBToolboxLibrary/wholeBodyModel/Jacobians/Jacobian  frameName=Frames.LEFT_FOOT
      settings: SourceProductName=Whole Body Toolbox
  Jacobian1 : WBToolboxLibrary/wholeBodyModel/Jacobians/Jacobian  frameName=Frames.RIGHT_FOOT
      settings: SourceProductName=Whole Body Toolbox
  References for H : MATLAB Function  TreatAsAtomicUnit=on
  Selector : Selector  InputPortWidth=6  IndexOptions=Index vector (dialog)  Indices=[4 5 6]  OutputSizes=1
  Sum : Sum  Inputs=|-+
  Switch : Switch  Criteria=u2 > Threshold  Threshold=0.1
  choose base to world transform : MATLAB Function  TreatAsAtomicUnit=on
  inertial : WBToolboxLibrary/Utilities/Yarp Read  portName=Ports.IMU  signalSize=12  timeout=0.5  blocking=off  timestamp=off  autoconnect=on  errorOnConnection=on
      settings: SourceProductName=Whole Body Toolbox
  intHw : Outport
  wires:
  qjDes/1 -> Jacobian/2, Sum/1, Jacobian1/2, Centroidal Momentum/2, Compute base to fixed link transform/1(qj)
  qj/1 -> Sum/2
  Sum/1 -> Centroidal Momentum/4, References for H/1(qjErr)
  References for H/1(nu_b_equivalent) -> Centroidal Momentum/3
  Jacobian/1 -> References for H/2(JL)
  Centroidal Momentum/1 -> Selector/1
  Selector/1 -> intHw/1
  Jacobian1/1 -> References for H/3(JR)
  constraints/1 -> References for H/4(activeFeetConstraints)
  state/1 -> choose base to world transform/1(state)
  choose base to world transform/1(booleanState) -> Switch/2
  Switch/1 -> Centroidal Momentum/1, Jacobian/1, Jacobian1/1
  inertial/1 -> Compute base to fixed link transform/2(inertial)
  Compute base to fixed link transform/1(fixed_LFoot_H_b) -> Switch/1
  Compute base to fixed link transform/2(fixed_RFoot_H_b) -> Switch/3

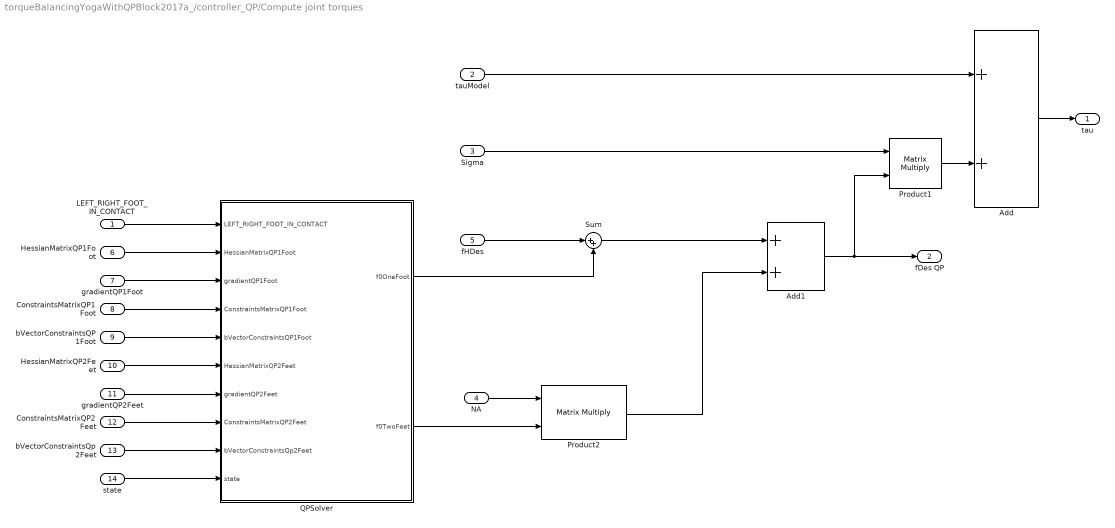
== system torqueBalancingYogaWithQPBlock2017a_/controller_QP/Compute joint torques ==
  LEFT_RIGHT_FOOT_IN_CONTACT : Inport
  tauModel : Inport  Port=2
  Sigma : Inport  Port=3
  NA : Inport  Port=4
  fHDes : Inport  Port=5
  HessianMatrixQP1Foot : Inport  Port=6
  gradientQP1Foot : Inport  Port=7
  ConstraintsMatrixQP1Foot : Inport  Port=8
  bVectorConstraintsQP1Foot : Inport  Port=9
  HessianMatrixQP2Feet : Inport  Port=10
  gradientQP2Feet : Inport  Port=11
  ConstraintsMatrixQP2Feet : Inport  Port=12
  bVectorConstraintsQp2Feet : Inport  Port=13
  state : Inport  Port=14
  Add : Sum
  Add1 : Sum
  Product1 : Product  Multiplication=Matrix(*)
  Product2 : Product  Multiplication=Matrix(*)
  QPSolver : Subsystem
  Sum : Sum  Inputs=|++
  "tau " : Outport
  fDes QP : Outport  Port=2
  wires:
  NA/1 -> Product2/1
  QPSolver/1(f0OneFoot) -> Sum/2
  Product1/1 -> Add/2
  tauModel/1 -> Add/1
  Add/1 -> "tau "/1
  Add1/1 -> fDes QP/1, Product1/2
  Sum/1 -> Add1/1
  Product2/1 -> Add1/2
  Sigma/1 -> Product1/1
  QPSolver/2(f0TwoFeet) -> Product2/2
  gradientQP1Foot/1 -> QPSolver/3(gradientQP1Foot)
  ConstraintsMatrixQP2Feet/1 -> QPSolver/8(ConstraintsMatrixQP2Feet)
  LEFT_RIGHT_FOOT_IN_CONTACT/1 -> QPSolver/1(LEFT_RIGHT_FOOT_IN_CONTACT)
  bVectorConstraintsQP1Foot/1 -> QPSolver/5(bVectorConstraintsQP1Foot)
  HessianMatrixQP1Foot/1 -> QPSolver/2(HessianMatrixQP1Foot)
  ConstraintsMatrixQP1Foot/1 -> QPSolver/4(ConstraintsMatrixQP1Foot)
  gradientQP2Feet/1 -> QPSolver/7(gradientQP2Feet)
  HessianMatrixQP2Feet/1 -> QPSolver/6(HessianMatrixQP2Feet)
  bVectorConstraintsQp2Feet/1 -> QPSolver/9(bVectorConstraintsQp2Feet)
  state/1 -> QPSolver/10(state)
  fHDes/1 -> Sum/1

== system torqueBalancingYogaWithQPBlock2017a_/controller_QP/Compute joint torques (motor reflected inertia) ==
  u : Inport
  " " : Constant  Value=Config.USE_MOTOR_REFLECTED_INERTIA
  "(transpose(T*Gamma))^{-1}*I_m*(T*Gamma)^{-1}" : MATLAB Function  TreatAsAtomicUnit=on
  Add : Sum  Inputs=-+
  Gain : Gain  Gain=Config.K_ff
  Get Measurement : WBToolboxLibrary/wholeBodyStates/Get Measurement  measuredType=Joints Acceleration
      settings: SourceProductName=Whole Body Toolbox
  Product : Product  Multiplication=Matrix(*)
  Switch : Switch  Criteria=u2 > Threshold
  tau_joints : Outport
  wires:
  Get Measurement/1 -> Product/2
  Product/1 -> Gain/1
  Gain/1 -> Add/1
  Add/1 -> Switch/1
  " "/1 -> Switch/2
  Switch/1 -> tau_joints/1
  u/1 -> Add/2, Switch/3
  "(transpose(T*Gamma))^{-1}*I_m*(T*Gamma)^{-1}"/1(reflectedInertia) -> Product/1

== system torqueBalancingYogaWithQPBlock2017a_/synchronizer/GAZEBO_SYNCHRONIZER ==
  Enable : EnablePort
  Simulator Synchronizer : WBToolboxLibrary/Utilities/Simulator Synchronizer  period=Config.Ts  serverPortName='/clock/rpc'  clientPortName='/WBT_synchronizer/rpc:o'
      settings: SourceProductName=Whole Body Toolbox

== system torqueBalancingYogaWithQPBlock2017a_/synchronizer/REAL_TIME_SYNC ==
  Enable : EnablePort
  Real Time Synchronizer : WBToolboxLibrary/Utilities/Real Time Synchronizer  period=Config.Ts
      settings: SourceProductName=Whole Body Toolbox

== system torqueBalancingYogaWithQPBlock2017a_/Dynamics and Kinematics/Dynamics/Add motors reflected inertias ==
  M : Inport
  Add motor reflected inertias : MATLAB Function  TreatAsAtomicUnit=on
  M_with_motor_inertia : Outport
  wires:
  M/1 -> Add motor reflected inertias/1(M)
  Add motor reflected inertias/1(M_with_inertia) -> M_with_motor_inertia/1

== system torqueBalancingYogaWithQPBlock2017a_/Dynamics and Kinematics/Kinematics/xCom ==
  w_H_b : Inport
  qj : Inport  Port=2
  CoM : WBToolboxLibrary/wholeBodyModel/Kinematics/Forward Kinematics  frameName=Frames.COM
      settings: SourceProductName=Whole Body Toolbox
  "CoM6D ->  CoMXYZ2" : Selector  NumberOfDimensions=2  InputPortWidth=7  IndexOptions=Index vector (dialog),Index vector (dialog)  Indices=[1 2 3],[4]  OutputSizes=1,1
  xCoM : Outport
  wires:
  qj/1 -> CoM/2
  "CoM6D ->  CoMXYZ2"/1 -> xCoM/1
  CoM/1 -> "CoM6D ->  CoMXYZ2"/1
  w_H_b/1 -> CoM/1

== system torqueBalancingYogaWithQPBlock2017a_/Robot State and References/Internal Coordinator/Base to fixed_link ==
  qj : Inport
  inertial : Inport  Port=2
  Constant1 : Constant  Value=Config.LEFT_FOOT_IN_CONTACT_AT_0
  Constant7 : Constant  Value=eye(4)
  "LFoot to base link transform " : Subsystem
  LFoot to world transform (fixed base) : WBToolboxLibrary/wholeBodyModel/Kinematics/Forward Kinematics  frameName=Frames.LEFT_FOOT
      settings: SourceProductName=Whole Body Toolbox
  RFoot to world transform (fixed base) : WBToolboxLibrary/wholeBodyModel/Kinematics/Forward Kinematics  frameName=Frames.RIGHT_FOOT
      settings: SourceProductName=Whole Body Toolbox
  Switch : Switch  Criteria=u2 > Threshold
  fixed_LFoot_H_b : Outport
  wires:
  "LFoot to base link transform "/1(link_H_b) -> fixed_LFoot_H_b/1
  inertial/1 -> "LFoot to base link transform "/2(inertial)
  qj/1 -> "LFoot to base link transform "/1(qj), RFoot to world transform (fixed base)/2, LFoot to world transform (fixed base)/2
  Constant7/1 -> LFoot to world transform (fixed base)/1, RFoot to world transform (fixed base)/1, "LFoot to base link transform "/4(w_H_base_fixed)
  Switch/1 -> "LFoot to base link transform "/3(w_H_link)
  LFoot to world transform (fixed base)/1 -> Switch/1
  RFoot to world transform (fixed base)/1 -> Switch/3
  Constant1/1 -> Switch/2

== system torqueBalancingYogaWithQPBlock2017a_/Robot State and References/Internal Coordinator/Compute State Velocity ==
  qj : Inport
  w_H_b : Inport  Port=2
  "feetInContact " : Inport  Port=3
  Compute Base Velocity : MATLAB Function  TreatAsAtomicUnit=on
  Feet Jacobians : Subsystem
  Get Measurement : WBToolboxLibrary/wholeBodyStates/Get Measurement  measuredType=Joints Velocity
      settings: SourceProductName=Whole Body Toolbox
  Mux : Mux  Inputs=2
  nu : Outport
  wires:
  Get Measurement/1 -> Mux/2, Compute Base Velocity/4(qjDot)
  Mux/1 -> nu/1
  "feetInContact "/1 -> Compute Base Velocity/3(feetInContact)
  Compute Base Velocity/1(nu_b) -> Mux/1
  qj/1 -> Feet Jacobians/1(qj)
  w_H_b/1 -> Feet Jacobians/2(w_H_b)
  Feet Jacobians/1(J_LFoot) -> Compute Base Velocity/1(J_LeftFoot)
  Feet Jacobians/2(J_RFoot) -> Compute Base Velocity/2(J_RightFoot)

== system torqueBalancingYogaWithQPBlock2017a_/Robot State and References/Internal Coordinator/xCom ==
  w_H_b : Inport
  qj : Inport  Port=2
  CoM : WBToolboxLibrary/wholeBodyModel/Kinematics/Forward Kinematics  frameName=Frames.COM
      settings: SourceProductName=Whole Body Toolbox
  "CoM6D ->  CoMXYZ2" : Selector  NumberOfDimensions=2  InputPortWidth=7  IndexOptions=Index vector (dialog),Index vector (dialog)  Indices=[1 2 3],[4]  OutputSizes=1,1
  xCoM : Outport
  wires:
  qj/1 -> CoM/2
  "CoM6D ->  CoMXYZ2"/1 -> xCoM/1
  CoM/1 -> "CoM6D ->  CoMXYZ2"/1
  w_H_b/1 -> CoM/1

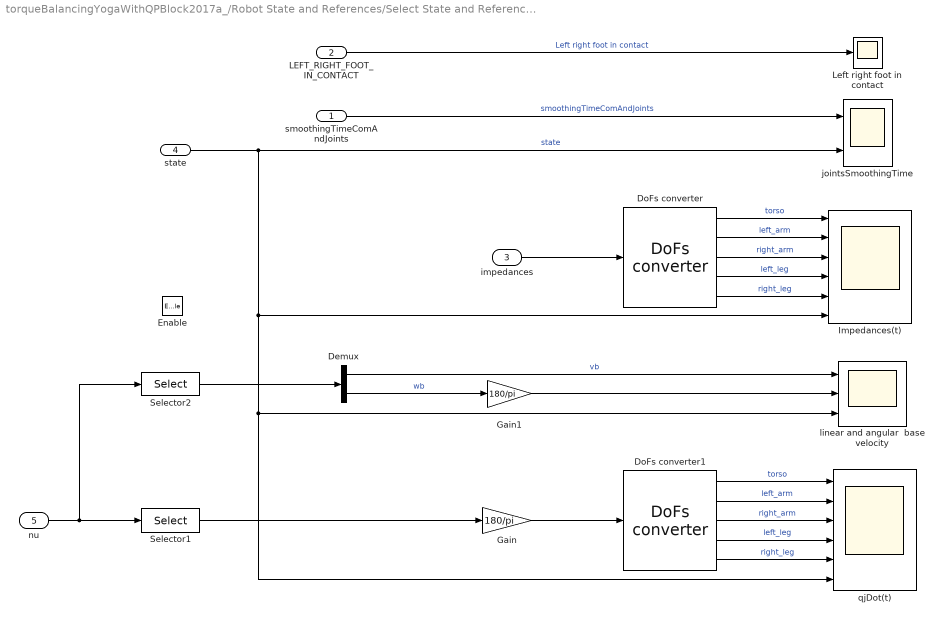
== system torqueBalancingYogaWithQPBlock2017a_/Robot State and References/Select State and References/Visualize Gain Tuning   ==
  smoothingTimeComAndJoints : Inport
  LEFT_RIGHT_FOOT_IN_CONTACT : Inport  Port=2
  impedances : Inport  Port=3
  state : Inport  Port=4
  nu : Inport  Port=5
  Enable : EnablePort
  Demux : Demux  Outputs=2
  DoFs converter : WBToolboxLibrary/Utilities/DoFs converter  yarp2WBIOption=From YARP to WBI
      settings: SourceProductName=Whole Body Toolbox
  DoFs converter1 : WBToolboxLibrary/Utilities/DoFs converter  yarp2WBIOption=From YARP to WBI
      settings: SourceProductName=Whole Body Toolbox
  Gain : Gain  Gain=180/pi
  Gain1 : Gain  Gain=180/pi
  Impedances(t) : Scope  NumInputPorts=6
  Left right foot in contact : Scope
  Selector1 : Selector  InputPortWidth=6+ROBOT_DOF  IndexOptions=Index vector (dialog)  Indices=[7:6+ROBOT_DOF]  OutputSizes=1
  Selector2 : Selector  InputPortWidth=6+ROBOT_DOF  IndexOptions=Index vector (dialog)  Indices=[1:6]  OutputSizes=1
  jointsSmoothingTime : Scope  NumInputPorts=2
  linear and angular  base velocity : Scope  NumInputPorts=3
  "qjDot(t) " : Scope  NumInputPorts=6
  wires:
  state/1 -> "qjDot(t) "/6, linear and angular  base velocity/3, Impedances(t)/6, jointsSmoothingTime/2  "state"
  LEFT_RIGHT_FOOT_IN_CONTACT/1 -> Left right foot in contact/1  "Left right foot in contact"
  impedances/1 -> DoFs converter/1
  smoothingTimeComAndJoints/1 -> jointsSmoothingTime/1  "smoothingTimeComAndJoints"
  DoFs converter/4 -> Impedances(t)/4  "left_leg"
  DoFs converter/5 -> Impedances(t)/5  "right_leg"
  DoFs converter/3 -> Impedances(t)/3  "right_arm"
  DoFs converter/1 -> Impedances(t)/1  "torso"
  DoFs converter/2 -> Impedances(t)/2  "left_arm"
  Selector1/1 -> Gain/1
  DoFs converter1/4 -> "qjDot(t) "/4  "left_leg"
  DoFs converter1/3 -> "qjDot(t) "/3  "right_arm"
  DoFs converter1/1 -> "qjDot(t) "/1  "torso"
  DoFs converter1/2 -> "qjDot(t) "/2  "left_arm"
  nu/1 -> Selector2/1, Selector1/1
  Selector2/1 -> Demux/1
  Demux/1 -> linear and angular  base velocity/1  "vb"
  Demux/2 -> Gain1/1  "wb"
  Gain/1 -> DoFs converter1/1
  Gain1/1 -> linear and angular  base velocity/2
  DoFs converter1/5 -> "qjDot(t) "/5  "right_leg"

== system torqueBalancingYogaWithQPBlock2017a_/Robot State and References/State Machine Yoga/Compute State Velocity ==
  qj : Inport
  w_H_b : Inport  Port=2
  "feetInContact " : Inport  Port=3
  Compute Base Velocity : MATLAB Function  TreatAsAtomicUnit=on
  Feet Jacobians : Subsystem
  Get Measurement : WBToolboxLibrary/wholeBodyStates/Get Measurement  measuredType=Joints Velocity
      settings: SourceProductName=Whole Body Toolbox
  Mux : Mux  Inputs=2
  nu : Outport
  wires:
  Get Measurement/1 -> Mux/2, Compute Base Velocity/4(qjDot)
  Mux/1 -> nu/1
  "feetInContact "/1 -> Compute Base Velocity/3(feetInContact)
  Compute Base Velocity/1(nu_b) -> Mux/1
  qj/1 -> Feet Jacobians/1(qj)
  w_H_b/1 -> Feet Jacobians/2(w_H_b)
  Feet Jacobians/1(J_LFoot) -> Compute Base Velocity/1(J_LeftFoot)
  Feet Jacobians/2(J_RFoot) -> Compute Base Velocity/2(J_RightFoot)

== system torqueBalancingYogaWithQPBlock2017a_/Robot State and References/State Machine Yoga/Compute base to fixed link transform ==
  qj : Inport
  inertial : Inport  Port=2
  Constant7 : Constant  Value=eye(4)
  "LFoot to base link transform " : Subsystem
  LFoot to world transform (fixed base) : WBToolboxLibrary/wholeBodyModel/Kinematics/Forward Kinematics  frameName=Frames.LEFT_FOOT
      settings: SourceProductName=Whole Body Toolbox
  RFoot to base link transform : Subsystem
  RFoot to world transform (fixed base) : WBToolboxLibrary/wholeBodyModel/Kinematics/Forward Kinematics  frameName=Frames.RIGHT_FOOT
      settings: SourceProductName=Whole Body Toolbox
  fixed_LFoot_H_b : Outport
  fixed_RFoot_H_b : Outport  Port=2
  wires:
  Constant7/1 -> RFoot to base link transform/4(w_H_base_fixed), "LFoot to base link transform "/4(w_H_base_fixed), RFoot to world transform (fixed base)/1, LFoot to world transform (fixed base)/1
  RFoot to base link transform/1(link_H_b) -> fixed_RFoot_H_b/1
  "LFoot to base link transform "/1(link_H_b) -> fixed_LFoot_H_b/1
  LFoot to world transform (fixed base)/1 -> "LFoot to base link transform "/3(w_H_link)
  RFoot to world transform (fixed base)/1 -> RFoot to base link transform/3(w_H_link)
  qj/1 -> "LFoot to base link transform "/1(qj), RFoot to base link transform/1(qj), RFoot to world transform (fixed base)/2, LFoot to world transform (fixed base)/2
  inertial/1 -> "LFoot to base link transform "/2(inertial), RFoot to base link transform/2(inertial)

== system torqueBalancingYogaWithQPBlock2017a_/Robot State and References/State Machine Yoga/Visualise extrnal wrenches   ==
  wL_WBDT : Inport
  wR_WBDT : Inport  Port=2
  Enable : EnablePort
  Constant : Constant  Value=Sm.wrench_thresholdContactOn
  Constant2 : Constant  Value=Sm.wrench_thresholdContactOff
  left foot ext wrench : Scope  NumInputPorts=3
  right foot ext wrench : Scope  NumInputPorts=3
  wires:
  Constant/1 -> left foot ext wrench/2, right foot ext wrench/2  "thresholdContactOn"
  wR_WBDT/1 -> right foot ext wrench/1  "wR_WBDT"
  wL_WBDT/1 -> left foot ext wrench/1  "wL_WBDT"
  Constant2/1 -> left foot ext wrench/3, right foot ext wrench/3  "thresholdContactOff"

== system torqueBalancingYogaWithQPBlock2017a_/Robot State and References/State Machine Yoga/xCom ==
  w_H_b : Inport
  qj : Inport  Port=2
  CoM : WBToolboxLibrary/wholeBodyModel/Kinematics/Forward Kinematics  frameName=Frames.COM
      settings: SourceProductName=Whole Body Toolbox
  "CoM6D ->  CoMXYZ2" : Selector  NumberOfDimensions=2  InputPortWidth=7  IndexOptions=Index vector (dialog),Index vector (dialog)  Indices=[1 2 3],[4]  OutputSizes=1,1
  xCoM : Outport
  wires:
  qj/1 -> CoM/2
  "CoM6D ->  CoMXYZ2"/1 -> xCoM/1
  CoM/1 -> "CoM6D ->  CoMXYZ2"/1
  w_H_b/1 -> CoM/1

== system torqueBalancingYogaWithQPBlock2017a_/Robot State and References/State Machine Yoga/xCom1 ==
  w_H_b : Inport
  qj : Inport  Port=2
  CoM : WBToolboxLibrary/wholeBodyModel/Kinematics/Forward Kinematics  frameName=Frames.COM
      settings: SourceProductName=Whole Body Toolbox
  "CoM6D ->  CoMXYZ2" : Selector  NumberOfDimensions=2  InputPortWidth=7  IndexOptions=Index vector (dialog),Index vector (dialog)  Indices=[1 2 3],[4]  OutputSizes=1,1
  xCoM : Outport
  wires:
  qj/1 -> CoM/2
  "CoM6D ->  CoMXYZ2"/1 -> xCoM/1
  CoM/1 -> "CoM6D ->  CoMXYZ2"/1
  w_H_b/1 -> CoM/1
